simulink model "P_1"  (R2019a)
settings: Solver=VariableStepAuto  StartTime=0.0  StopTime=10.0  RelTol=1e-3
settings Model: Creator=john  LastModifiedBy=john

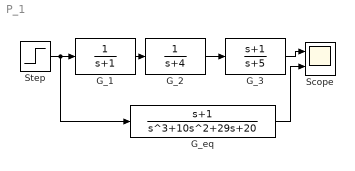
== system P_1 ==
  G_1 : TransferFcn  Denominator=[1 1]
  "G_2 " : TransferFcn  Denominator=[1 4]
  G_3 : TransferFcn  Numerator=[1 1]  Denominator=[1 5]
  G_eq : TransferFcn  Numerator=[1 1]  Denominator=[1 10 29 20]
  Scope : Scope  NumInputPorts=2
  Step : Step  SampleTime=0
  wires:
  "G_2 "/1 -> G_3/1
  G_1/1 -> "G_2 "/1
  Step/1 -> G_eq/1, G_1/1
  G_3/1 -> Scope/1
  G_eq/1 -> Scope/2
